simulink model "MMC_9lvl_matriz_tri_v12_Renner"  (R2025a)
settings: Solver=FixedStepAuto  StartTime=0.0  StopTime=5  FixedStep=0.0000005  MaxStep=1e-6  RelTol=1e-3
InitFcn:
  | C=4000e-6;
  | Larm=15e-3;
  | Rarm=0;
  | R=5;
  | L=100e-6;
  | Vcc=250;
  | Vsm=Vcc*2/4;
  | Vcap0=Vsm;
  | FR=20000;
  | TS=1/FR; %0.00005 = 50 microsec
  | Vsa=120;
  | Pref=3000;
  | Qref=0;
libraries: spsIGBTDiodeLib x48, spsVoltageMeasurementLib x34, spsSeriesRLCBranchLib x33, spsCurrentMeasurementLib x10, spsGroundLib x4, spsACVoltageSourceLib x3, SignalEditorBlockLib x2, spsDCVoltageSourceLib x2, spsPowerLib x1, sps_lib x1
(part 1 of 2)
settings Model: Creator=bernardo  LastModifiedBy=renner
settings SolverCC: ZeroCrossAlgorithm=Adaptive  AlgebraicLoopSolver=TrustRegion
settings DataIOCC: ReturnWorkspaceOutputs=off
settings OptimizationCC: ReuseModelBlockBuffer=off
settings DebuggingCC: IgnoredZcDiagnostic=none  UnconnectedInputMsg=warning  UnconnectedOutputMsg=warning  UnconnectedLineMsg=warning  ArithmeticOperatorsInVariantConditions=warning
settings ModelReferenceCC: EnableRefExpFcnMdlSchedulingChecks=on
settings SFSimCC: SimUseLocalCustomCode=off  CustomCodeUndefinedFunction=UseInterfaceOnly
settings RTWCC: RTWUseLocalCustomCode=off  GPUComputeCapability=3.5

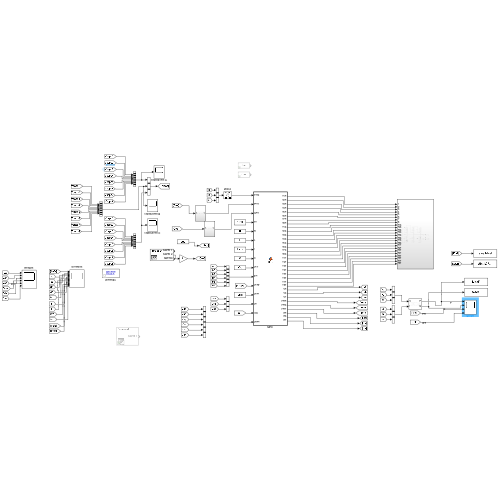
[thumbnail: Simulink's stored preview of the top-level diagram]
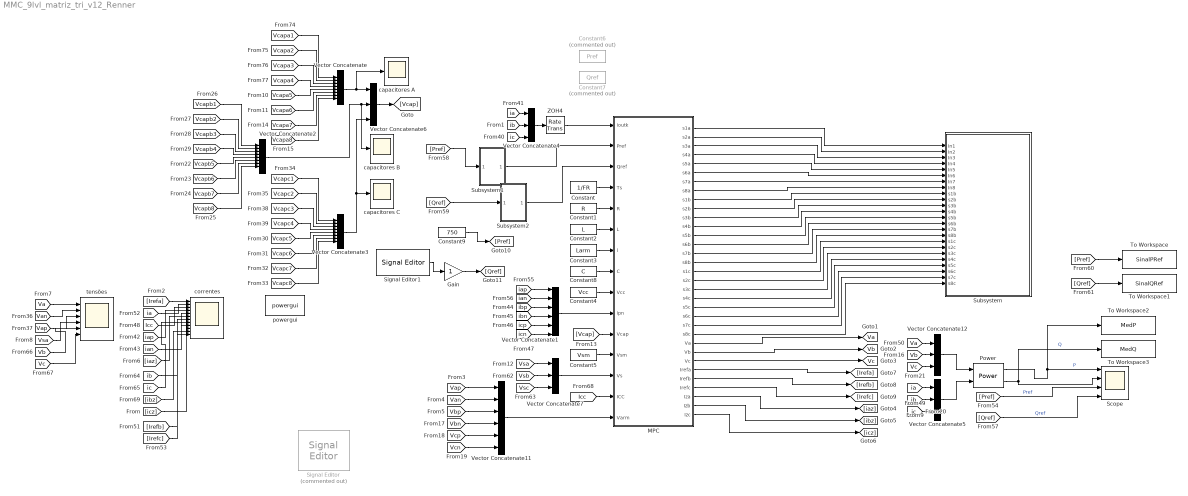
== system MMC_9lvl_matriz_tri_v12_Renner ==
  Constant : Constant  Value=1/FR
  Constant1 : Constant  Value=R
  Constant2 : Constant  Value=L
  Constant3 : Constant  Value=Larm
  Constant4 : Constant  Value=Vcc
  Constant5 : Constant  Value=Vsm
  Constant6 : Constant  Commented=on  Value=Pref
  Constant7 : Constant  Commented=on  Value=Qref
  Constant8 : Constant  Value=C
  Constant9 : Constant  Value=750
  Gain : Gain
  MPC : MATLAB Function  TreatAsAtomicUnit=on  SystemSampleTime=0.00005
  Power : spsPowerLib/Power  Freq=60  Vinit=[1, 0]  Iinit=[1, 0]  Ts=0
  Scope : Scope  NumInputPorts=4
      settings: ActiveDisplayYMinimum=-323.77012117483849  ActiveDisplayYMaximum=2913.931090573547
  Signal Editor : SignalEditorBlockLib/Signal Editor  Commented=on  FileName=G:\My Drive\PESQUISA\SIMULACOES\sinais.mat  ActiveScenario=Scenario2  ActiveSignal=Steps Q  IsBus=off  OutputBusObjectStr=Bus: BusObject  SampleTime=0  Interpolate=off  ZeroCross=off  OutputAfterFinalValue=Setting to zero  Unit=inherit  PreserveSignalName=on  ApplySigPropsToAllScenarios=on  ApplySigPropsToAllSignals=on  SignalPropertySource=Dialog parameters
  Signal Editor1 : SignalEditorBlockLib/Signal Editor  FileName=/Users/renner/Downloads/Sinais.mat  ActiveScenario=Scenario  ActiveSignal=Signal 2  IsBus=off  OutputBusObjectStr=Bus: BusObject  SampleTime=0  ZeroCross=off  OutputAfterFinalValue=Setting to zero  Unit=inherit  PreserveSignalName=on  ApplySigPropsToAllScenarios=on  ApplySigPropsToAllSignals=off  SignalPropertySource=Dialog parameters
  Subsystem : Subsystem
  Subsystem1 : Subsystem
  Subsystem2 : Subsystem
  To Workspace : ToWorkspace  VariableName=SinalPRef  SampleTime=0.0005
      settings: Decimation=3  Save2DSignal=2-D array (concatenate along first dimension)
  To Workspace1 : ToWorkspace  VariableName=SinalQRef  SampleTime=0.0005
      settings: Decimation=3  Save2DSignal=2-D array (concatenate along first dimension)
  To Workspace2 : ToWorkspace  VariableName=MedP  SampleTime=0.0005
      settings: Decimation=3  Save2DSignal=2-D array (concatenate along first dimension)
  To Workspace3 : ToWorkspace  VariableName=MedQ  SampleTime=0.0005
      settings: Decimation=3  Save2DSignal=2-D array (concatenate along first dimension)
  Vector Concatenate : Concatenate  NumInputs=8
  Vector Concatenate1 : Concatenate  NumInputs=6
  Vector Concatenate11 : Concatenate  NumInputs=6
  Vector Concatenate{4..7,12} (5 alike) : Concatenate  NumInputs=3
  Vector Concatenate2 : Concatenate  NumInputs=8
  Vector Concatenate3 : Concatenate  NumInputs=8
  ZOH4 : RateTransition  OutPortSampleTime=TS
  capacitores A : Scope
      settings: ActiveDisplayYMinimum=96.83935  ActiveDisplayYMaximum=130.64864
  capacitores B : Scope
      settings: ActiveDisplayYMinimum=97.09716  ActiveDisplayYMaximum=129.55775  DataLoggingVariableName=ScopeData2
  capacitores C : Scope
      settings: ActiveDisplayYMinimum=97.83131  ActiveDisplayYMaximum=129.00851  DataLoggingVariableName=ScopeData3
  correntes : Scope  NumInputPorts=12
      settings: ActiveDisplayYMinimum=-28.003686399512119  ActiveDisplayYMaximum=28.003686399512119
  powergui : sps_lib/powergui  Priority=1  SimulationMode=Discrete  SampleTime=0.00005  frequency=60  Iterations=50  frequencyindice=0  Pbase=100e6  ErrMax=1e-4  UnitsV=kV  UnitsW=MW  buscounter=0  FunctionMessages=off  echomessages=off  EnableUseOfTLC=off  CurrentSourceSwitches=off  DisableSnubberDevices=off  DisableRonSwitches=off  DisableVfSwitches=off  DisplayEquations=off  AutomaticDiscreteSolvers=off  SolverType=Tustin/Backward Euler (TBE)  Interpol=off  ExternalGateDelay=off  methode=off  Ts=100  x0status=blocks  SPID=on  SwTol=0  HookPort=off  NonlinearTolerance=1e-4  nMaxIteration=100  ContinueOnMaxIteration=off  RestoreLinks=warning  ResistiveCurrentMeasurement=off  Frange=[0:2:500]  Ylog=off  Xlog=on  ShowGrid=off  save=off  variable=ZData  structure=Scope1  ZoomFFT=off  StartTime=0.0  cycles=10  DisplayStyle=2  fundamental=60  FreqAxis=off  MaxFrequency=20000  frequencyindicesteady=1  RmsSteady=1  display=off
  tensões : Scope  NumInputPorts=6
      settings: ActiveDisplayYMinimum=-296.50571696969695  ActiveDisplayYMaximum=516.307633030303  DataLoggingVariableName=ScopeData2
  tag scope: Va=global, Vb=global, Vc=global
  wires:
  Constant1/1 -> MPC/5(R)
  Constant/1 -> MPC/4(Ts)
  Constant3/1 -> MPC/7(l)
  Constant4/1 -> MPC/9(Vcc)
  Constant2/1 -> MPC/6(L)
  [iap] -> correntes/4
  [ian] -> correntes/5
  [Icc] -> correntes/3
  [ia] -> correntes/2
  [Van] -> tensões/2
  [Vcapa1] -> Vector Concatenate/1
  [Vcapa2] -> Vector Concatenate/2
  [Vcapa3] -> Vector Concatenate/3
  [Vcapa4] -> Vector Concatenate/4
  [iap] -> Vector Concatenate1/1
  [ian] -> Vector Concatenate1/2
  Vector Concatenate1/1 -> MPC/10(ipn)
  [Vap] -> tensões/3
  [Vcapa5] -> Vector Concatenate/5
  [Vcapa6] -> Vector Concatenate/6
  [Vcapa7] -> Vector Concatenate/7
  [Vcapa8] -> Vector Concatenate/8
  [Irefa] -> correntes/1
  [iaz] -> correntes/6
  MPC/1(s1a) -> Subsystem/1(In1)
  MPC/2(s2a) -> Subsystem/2(In2)
  MPC/3(s3a) -> Subsystem/3(In3)
  MPC/4(s4a) -> Subsystem/4(In4)
  MPC/5(s5a) -> Subsystem/5(In5)
  MPC/6(s6a) -> Subsystem/6(In6)
  MPC/7(s7a) -> Subsystem/7(In7)
  MPC/8(s8a) -> Subsystem/8(In8)
  Constant5/1 -> MPC/12(Vsm)
  [Vsa] -> tensões/4
  [Va] -> tensões/1
  [Vcap] -> MPC/11(Vcap)
  Vector Concatenate2/1 -> capacitores B/1, Vector Concatenate6/2
  [Vcapb7] -> Vector Concatenate2/7
  [Vcapb5] -> Vector Concatenate2/5
  [Vcapb6] -> Vector Concatenate2/6
  [Vcapb3] -> Vector Concatenate2/3
  [Vcapb1] -> Vector Concatenate2/1
  [Vcapb2] -> Vector Concatenate2/2
  [Vcapb8] -> Vector Concatenate2/8
  [Vcapb4] -> Vector Concatenate2/4
  [Vcapc6] -> Vector Concatenate3/6
  [Vcapc4] -> Vector Concatenate3/4
  [Vcapc3] -> Vector Concatenate3/3
  [Vcapc1] -> Vector Concatenate3/1
  [Vcapc2] -> Vector Concatenate3/2
  [Vcapc8] -> Vector Concatenate3/8
  [Vcapc5] -> Vector Concatenate3/5
  Vector Concatenate3/1 -> Vector Concatenate6/3, capacitores C/1
  [Vcapc7] -> Vector Concatenate3/7
  MPC/9(s1b) -> Subsystem/9(s1b)
  MPC/10(s2b) -> Subsystem/10(s2b)
  MPC/11(s3b) -> Subsystem/11(s3b)
  MPC/12(s4b) -> Subsystem/12(s4b)
  MPC/13(s5b) -> Subsystem/13(s5b)
  MPC/14(s6b) -> Subsystem/14(s6b)
  MPC/15(s7b) -> Subsystem/15(s7b)
  MPC/16(s8b) -> Subsystem/16(s8b)
  MPC/17(s1c) -> Subsystem/17(s1c)
  MPC/18(s2c) -> Subsystem/18(s2c)
  MPC/19(s3c) -> Subsystem/19(s3c)
  MPC/20(s4c) -> Subsystem/20(s4c)
  MPC/21(s5c) -> Subsystem/21(s5c)
  MPC/22(s6c) -> Subsystem/22(s6c)
  MPC/23(s7c) -> Subsystem/23(s7c)
  MPC/24(s8c) -> Subsystem/24(s8c)
  [ia] -> Vector Concatenate4/1
  [ib] -> Vector Concatenate4/2
  [ic] -> Vector Concatenate4/3
  Vector Concatenate4/1 -> ZOH4/1
  ZOH4/1 -> MPC/1(ioutk)
  [ibp] -> Vector Concatenate1/3
  [ibn] -> Vector Concatenate1/4
  [icp] -> Vector Concatenate1/5
  [icn] -> Vector Concatenate1/6
  Vector Concatenate/1 -> capacitores A/1, Vector Concatenate6/1
  Vector Concatenate6/1 -> [Vcap]
  [Vsc] -> Vector Concatenate7/3
  [ib] -> correntes/7
  [ic] -> correntes/8
  [Vb] -> tensões/5
  [Vc] -> tensões/6
  [Icc] -> MPC/14(ICC)
  [ibz] -> correntes/9
  [icz] -> correntes/10
  [Vap] -> Vector Concatenate11/1
  [Van] -> Vector Concatenate11/2
  [Vbp] -> Vector Concatenate11/3
  [Vbn] -> Vector Concatenate11/4
  [Vcp] -> Vector Concatenate11/5
  [Vcn] -> Vector Concatenate11/6
  Vector Concatenate11/1 -> MPC/15(Varm)
  Vector Concatenate7/1 -> MPC/13(Vs)
  [Vsa] -> Vector Concatenate7/1
  [Vsb] -> Vector Concatenate7/2
  MPC/25(Va) -> [Va]
  MPC/26(Vb) -> [Vb]
  MPC/27(Vc) -> [Vc]
  MPC/28(Irefa) -> [Irefa]
  MPC/29(Irefb) -> [Irefb]
  MPC/30(Irefc) -> [Irefc]
  MPC/31(Iza) -> [iaz]
  MPC/32(Izb) -> [ibz]
  MPC/33(Izc) -> [icz]
  [ia] -> Vector Concatenate5/1
  [ic] -> Vector Concatenate5/3
  [Vb] -> Vector Concatenate12/2
  [Vc] -> Vector Concatenate12/3
  [Va] -> Vector Concatenate12/1
  [ib] -> Vector Concatenate5/2
  [Irefb] -> correntes/11
  [Irefc] -> correntes/12
  Constant8/1 -> MPC/8(C)
  Power/1 -> Scope/1, To Workspace2/1  "P"
  Power/2 -> Scope/2, To Workspace3/1  "Q"
  Vector Concatenate12/1 -> Power/1
  Vector Concatenate5/1 -> Power/2
  [Qref] -> Subsystem2/1(In1)
  [Pref] -> To Workspace/1
  [Qref] -> To Workspace1/1
  [Pref] -> Subsystem1/1(In1)
  Subsystem1/1(Out1) -> MPC/2(Pref)
  [Pref] -> Scope/3  "Pref"
  Constant9/1 -> [Pref]
  [Qref] -> Scope/4  "Qref"
  Gain/1 -> [Qref]
  Subsystem2/1(Out1) -> MPC/3(Qref)
  Signal Editor1/2 -> Gain/1

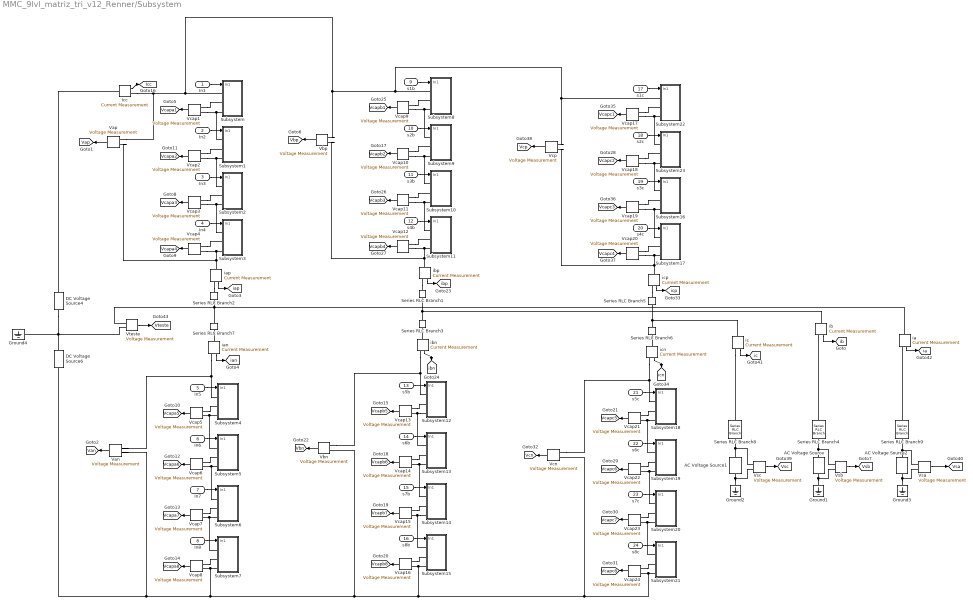
== system MMC_9lvl_matriz_tri_v12_Renner/Subsystem ==
  In1 : Inport
  In2 : Inport  Port=2
  In3 : Inport  Port=3
  In4 : Inport  Port=4
  In5 : Inport  Port=5
  In6 : Inport  Port=6
  In7 : Inport  Port=7
  In8 : Inport  Port=8
  s1b : Inport  Port=9
  s2b : Inport  Port=10
  s3b : Inport  Port=11
  s4b : Inport  Port=12
  s5b : Inport  Port=13
  s6b : Inport  Port=14
  s7b : Inport  Port=15
  s8b : Inport  Port=16
  s1c : Inport  Port=17
  s2c : Inport  Port=18
  s3c : Inport  Port=19
  s4c : Inport  Port=20
  s5c : Inport  Port=21
  s6c : Inport  Port=22
  s7c : Inport  Port=23
  s8c : Inport  Port=24
  AC Voltage Source : spsACVoltageSourceLib/AC Voltage Source  Amplitude=Vsa  Phase=-120  Frequency=60  SampleTime=0  Measurements=None  BusType=swing  Pref=10e3  Qref=0  Qmin=-inf  Qmax=+inf
  AC Voltage Source1 : spsACVoltageSourceLib/AC Voltage Source  Amplitude=Vsa  Phase=120  Frequency=60  SampleTime=0  Measurements=None  BusType=swing  Pref=10e3  Qref=0  Qmin=-inf  Qmax=+inf
  AC Voltage Source2 : spsACVoltageSourceLib/AC Voltage Source  Amplitude=Vsa  Phase=0  Frequency=60  SampleTime=0  Measurements=None  BusType=swing  Pref=10e3  Qref=0  Qmin=-inf  Qmax=+inf
  DC Voltage Source4 : spsDCVoltageSourceLib/DC Voltage Source  Amplitude=Vcc  Measurements=None
  DC Voltage Source6 : spsDCVoltageSourceLib/DC Voltage Source  Amplitude=Vcc  Measurements=None
  Ground{1..4} (4 alike) : spsGroundLib/Ground  LConnTagsString=a
  Icc : spsCurrentMeasurementLib/Current Measurement  PhasorSimulation=off  OutputType=Magnitude  PSBequivalent=0
  Series RLC Branch{1..3,5..7} (6 alike) : spsSeriesRLCBranchLib/Series RLC Branch  LConnTagsString=__new0  RConnTagsString=__new0  BranchType=L  Resistance=0  Inductance=Larm  SetiL0=off  InitialCurrent=0  Capacitance=0  Setx0=off  InitialVoltage=0  Measurements=None
  Series RLC Branch4 : spsSeriesRLCBranchLib/Series RLC Branch  LConnTagsString=__new0  RConnTagsString=__new0  BranchType=RL  Resistance=R  Inductance=L  SetiL0=off  InitialCurrent=0  Capacitance=1e-6  Setx0=off  InitialVoltage=0  Measurements=None
  Series RLC Branch8 : spsSeriesRLCBranchLib/Series RLC Branch  LConnTagsString=__new0  RConnTagsString=__new0  BranchType=RL  Resistance=R  Inductance=L  SetiL0=off  InitialCurrent=0  Capacitance=1e-6  Setx0=off  InitialVoltage=0  Measurements=None
  Series RLC Branch9 : spsSeriesRLCBranchLib/Series RLC Branch  LConnTagsString=__new0  RConnTagsString=__new0  BranchType=RL  Resistance=R  Inductance=L  SetiL0=off  InitialCurrent=0  Capacitance=1e-6  Setx0=off  InitialVoltage=0  Measurements=None
  Subsystem : Subsystem
  Subsystem1 : Subsystem
  Subsystem10 : Subsystem
  Subsystem11 : Subsystem
  Subsystem12 : Subsystem
  Subsystem13 : Subsystem
  Subsystem14 : Subsystem
  Subsystem15 : Subsystem
  Subsystem16 : Subsystem
  Subsystem17 : Subsystem
  Subsystem18 : Subsystem
  Subsystem19 : Subsystem
  Subsystem2 : Subsystem
  Subsystem20 : Subsystem
  Subsystem21 : Subsystem
  Subsystem22 : Subsystem
  Subsystem23 : Subsystem
  Subsystem3 : Subsystem
  Subsystem4 : Subsystem
  Subsystem5 : Subsystem
  Subsystem6 : Subsystem
  Subsystem7 : Subsystem
  Subsystem8 : Subsystem
  Subsystem9 : Subsystem
  Van : spsVoltageMeasurementLib/Voltage Measurement  PhasorSimulation=off  OutputType=Complex  PSBequivalent=0
  Vap : spsVoltageMeasurementLib/Voltage Measurement  PhasorSimulation=off  OutputType=Complex  PSBequivalent=0
  Vbn : spsVoltageMeasurementLib/Voltage Measurement  PhasorSimulation=off  OutputType=Complex  PSBequivalent=0
  Vbp : spsVoltageMeasurementLib/Voltage Measurement  PhasorSimulation=off  OutputType=Complex  PSBequivalent=0
  Vcap{1..24} (24 alike) : spsVoltageMeasurementLib/Voltage Measurement  PhasorSimulation=off  OutputType=Complex  PSBequivalent=0
  Vcn : spsVoltageMeasurementLib/Voltage Measurement  PhasorSimulation=off  OutputType=Complex  PSBequivalent=0
  Vcp : spsVoltageMeasurementLib/Voltage Measurement  PhasorSimulation=off  OutputType=Complex  PSBequivalent=0
  Vsa : spsVoltageMeasurementLib/Voltage Measurement  PhasorSimulation=off  OutputType=Complex  PSBequivalent=0
  Vsb : spsVoltageMeasurementLib/Voltage Measurement  PhasorSimulation=off  OutputType=Complex  PSBequivalent=0
  Vsc : spsVoltageMeasurementLib/Voltage Measurement  PhasorSimulation=off  OutputType=Complex  PSBequivalent=0
  Vteste : spsVoltageMeasurementLib/Voltage Measurement  PhasorSimulation=off  OutputType=Complex  PSBequivalent=0
  ia : spsCurrentMeasurementLib/Current Measurement  PhasorSimulation=off  OutputType=Magnitude  PSBequivalent=0
  ian : spsCurrentMeasurementLib/Current Measurement  PhasorSimulation=off  OutputType=Magnitude  PSBequivalent=0
  iap : spsCurrentMeasurementLib/Current Measurement  PhasorSimulation=off  OutputType=Magnitude  PSBequivalent=0
  ib : spsCurrentMeasurementLib/Current Measurement  PhasorSimulation=off  OutputType=Magnitude  PSBequivalent=0
  ibn : spsCurrentMeasurementLib/Current Measurement  PhasorSimulation=off  OutputType=Magnitude  PSBequivalent=0
  ibp : spsCurrentMeasurementLib/Current Measurement  PhasorSimulation=off  OutputType=Magnitude  PSBequivalent=0
  ic : spsCurrentMeasurementLib/Current Measurement  PhasorSimulation=off  OutputType=Magnitude  PSBequivalent=0
  icn : spsCurrentMeasurementLib/Current Measurement  PhasorSimulation=off  OutputType=Magnitude  PSBequivalent=0
  icp : spsCurrentMeasurementLib/Current Measurement  PhasorSimulation=off  OutputType=Magnitude  PSBequivalent=0
  tag scope: Icc=global, Van=global, Vap=global, Vbn=global, Vbp=global, Vcapa1=global, Vcapa2=global, Vcapa3=global, Vcapa4=global, Vcapa5=global, Vcapa6=global, Vcapa7=global, Vcapa8=global, Vcapb1=global, Vcapb2=global, Vcapb3=global, Vcapb4=global, Vcapb5=global, Vcapb6=global, Vcapb7=global, Vcapb8=global, Vcapc1=global, Vcapc2=global, Vcapc3=global, Vcapc4=global, Vcapc5=global, Vcapc6=global, Vcapc7=global, Vcapc8=global, Vcn=global, Vcp=global, Vsa=global, Vsb=global, Vsc=global, Vteste=global, ia=global, ian=global, iap=global, ib=global, ibn=global, ibp=global, ic=global, icn=global, icp=global
  wires:
  ib/1 -> [ib]
  Van/1 -> [Van]
  iap/1 -> [iap]
  ian/1 -> [ian]
  Vcap1/1 -> [Vcapa1]
  In1/1 -> Subsystem/1(In1)
  In2/1 -> Subsystem1/1(In1)
  Vcap2/1 -> [Vcapa2]
  Vcap3/1 -> [Vcapa3]
  In3/1 -> Subsystem2/1(In1)
  In4/1 -> Subsystem3/1(In1)
  Vcap4/1 -> [Vcapa4]
  In5/1 -> Subsystem4/1(In1)
  Vcap5/1 -> [Vcapa5]
  Vap/1 -> [Vap]
  Vcap6/1 -> [Vcapa6]
  In6/1 -> Subsystem5/1(In1)
  In8/1 -> Subsystem7/1(In1)
  Vcap8/1 -> [Vcapa8]
  Vcap7/1 -> [Vcapa7]
  In7/1 -> Subsystem6/1(In1)
  Icc/1 -> [Icc]
  Vsb/1 -> [Vsb]
  s6b/1 -> Subsystem13/1(In1)
  s5b/1 -> Subsystem12/1(In1)
  ibn/1 -> [ibn]
  Vcap12/1 -> [Vcapb4]
  Vcap16/1 -> [Vcapb8]
  s2b/1 -> Subsystem9/1(In1)
  s8b/1 -> Subsystem15/1(In1)
  Vcap13/1 -> [Vcapb5]
  ibp/1 -> [ibp]
  Vcap10/1 -> [Vcapb2]
  s4b/1 -> Subsystem11/1(In1)
  s7b/1 -> Subsystem14/1(In1)
  Vbp/1 -> [Vbp]
  s1b/1 -> Subsystem8/1(In1)
  s3b/1 -> Subsystem10/1(In1)
  Vbn/1 -> [Vbn]
  Vcap14/1 -> [Vcapb6]
  Vcap9/1 -> [Vcapb1]
  Vcap15/1 -> [Vcapb7]
  Vcap11/1 -> [Vcapb3]
  Vcap19/1 -> [Vcapc3]
  Vcap22/1 -> [Vcapc6]
  s3c/1 -> Subsystem16/1(In1)
  Vcap23/1 -> [Vcapc7]
  Vcp/1 -> [Vcp]
  Vcap21/1 -> [Vcapc5]
  s7c/1 -> Subsystem20/1(In1)
  Vcap17/1 -> [Vcapc1]
  s6c/1 -> Subsystem19/1(In1)
  icn/1 -> [icn]
  s8c/1 -> Subsystem21/1(In1)
  s2c/1 -> Subsystem23/1(In1)
  s5c/1 -> Subsystem18/1(In1)
  s4c/1 -> Subsystem17/1(In1)
  icp/1 -> [icp]
  Vcap18/1 -> [Vcapc2]
  Vcap20/1 -> [Vcapc4]
  Vcap24/1 -> [Vcapc8]
  s1c/1 -> Subsystem22/1(In1)
  Vcn/1 -> [Vcn]
  Vsc/1 -> [Vsc]
  Vsa/1 -> [Vsa]
  ia/1 -> [ia]
  ic/1 -> [ic]
  Vteste/1 -> [Vteste]
  connections:
  Vcap1/LConn2 -- Subsystem1/LConn1 -- Subsystem/LConn3
  Vcap1/LConn1 -- Subsystem/LConn2
  Vcap2/LConn1 -- Subsystem1/LConn2
  Vcap2/LConn2 -- Subsystem2/LConn1 -- Subsystem1/LConn3
  Vcap3/LConn2 -- Subsystem3/LConn1 -- Subsystem2/LConn3
  Vcap3/LConn1 -- Subsystem2/LConn2
  Vcap4/LConn2 -- Vap/LConn2 -- iap/LConn1 -- Subsystem3/LConn3
  Vcap4/LConn1 -- Subsystem3/LConn2
  Icc/LConn1 -- DC Voltage Source4/RConn1
  iap/RConn1 -- Series RLC Branch2/RConn1
  Series RLC Branch7/RConn1 -- Vteste/LConn1 -- ia/LConn1 -- Series RLC Branch2/LConn1
  Series RLC Branch4/LConn1 -- ib/RConn1
  ian/LConn1 -- Series RLC Branch7/LConn1
  ian/RConn1 -- Van/LConn1 -- Subsystem4/LConn1
  Vcap5/LConn2 -- Subsystem5/LConn1 -- Subsystem4/LConn3
  Vcap5/LConn1 -- Subsystem4/LConn2
  Vcap6/LConn1 -- Subsystem5/LConn2
  Vcap6/LConn2 -- Subsystem6/LConn1 -- Subsystem5/LConn3
  Subsystem7/LConn1 -- Vcap7/LConn2 -- Subsystem6/LConn3
  Subsystem21/LConn3 -- Vcap24/LConn2 -- Vbn/LConn2 -- DC Voltage Source6/LConn1 -- Van/LConn2 -- Vcap8/LConn2 -- Subsystem7/LConn3 -- Vcap16/LConn2 -- Subsystem15/LConn3 -- Vcn/LConn2
  Vcap8/LConn1 -- Subsystem7/LConn2
  Vcap7/LConn1 -- Subsystem6/LConn2
  Vcp/LConn1 -- Vbp/LConn1 -- Vap/LConn1 -- Icc/RConn1 -- Subsystem/LConn1 -- Subsystem8/LConn1 -- Subsystem22/LConn1
  Ground4/LConn1 -- DC Voltage Source4/LConn1 -- Vteste/LConn2 -- DC Voltage Source6/RConn1
  AC Voltage Source/RConn1 -- Vsb/LConn1 -- Series RLC Branch4/RConn1
  Ground1/LConn1 -- AC Voltage Source/LConn1 -- Vsb/LConn2
  Subsystem10/LConn3 -- Vcap11/LConn2 -- Subsystem11/LConn1
  Subsystem11/LConn3 -- Vcap12/LConn2 -- Vbp/LConn2 -- ibp/LConn1
  Subsystem12/LConn1 -- ibn/RConn1 -- Vbn/LConn1
  Subsystem12/LConn3 -- Vcap13/LConn2 -- Subsystem13/LConn1
  Series RLC Branch3/RConn1 -- ib/LConn1 -- Series RLC Branch1/LConn1
  Subsystem9/LConn3 -- Vcap10/LConn2 -- Subsystem10/LConn1
  Subsystem8/LConn3 -- Vcap9/LConn2 -- Subsystem9/LConn1
  Subsystem13/LConn3 -- Vcap14/LConn2 -- Subsystem14/LConn1
  Subsystem14/LConn3 -- Subsystem15/LConn1 -- Vcap15/LConn2
  Vcap11/LConn1 -- Subsystem10/LConn2
  Vcap15/LConn1 -- Subsystem14/LConn2
  ibn/LConn1 -- Series RLC Branch3/LConn1
  ibp/RConn1 -- Series RLC Branch1/RConn1
  Vcap12/LConn1 -- Subsystem11/LConn2
  Vcap9/LConn1 -- Subsystem8/LConn2
  Vcap10/LConn1 -- Subsystem9/LConn2
  Vcap14/LConn1 -- Subsystem13/LConn2
  Vcap16/LConn1 -- Subsystem15/LConn2
  Vcap13/LConn1 -- Subsystem12/LConn2
  Subsystem19/LConn3 -- Vcap22/LConn2 -- Subsystem20/LConn1
  Subsystem22/LConn3 -- Vcap17/LConn2 -- Subsystem23/LConn1
  Subsystem20/LConn3 -- Subsystem21/LConn1 -- Vcap23/LConn2
  ic/RConn1 -- Series RLC Branch8/LConn1
  Subsystem18/LConn3 -- Vcap21/LConn2 -- Subsystem19/LConn1
  Subsystem18/LConn1 -- icn/RConn1 -- Vcn/LConn1
  Subsystem17/LConn3 -- Vcap20/LConn2 -- Vcp/LConn2 -- icp/LConn1
  Subsystem16/LConn3 -- Vcap19/LConn2 -- Subsystem17/LConn1
  Subsystem23/LConn3 -- Vcap18/LConn2 -- Subsystem16/LConn1
  Vcap21/LConn1 -- Subsystem18/LConn2
  Vcap18/LConn1 -- Subsystem23/LConn2
  Vcap24/LConn1 -- Subsystem21/LConn2
  Vcap17/LConn1 -- Subsystem22/LConn2
  Vcap22/LConn1 -- Subsystem19/LConn2
  Vcap20/LConn1 -- Subsystem17/LConn2
  Vcap23/LConn1 -- Subsystem20/LConn2
  icn/LConn1 -- Series RLC Branch6/LConn1
  icp/RConn1 -- Series RLC Branch5/RConn1
  Vcap19/LConn1 -- Subsystem16/LConn2
  AC Voltage Source1/RConn1 -- Vsc/LConn1 -- Series RLC Branch8/RConn1
  Ground2/LConn1 -- AC Voltage Source1/LConn1 -- Vsc/LConn2
  AC Voltage Source2/RConn1 -- Vsa/LConn1 -- Series RLC Branch9/RConn1
  Ground3/LConn1 -- AC Voltage Source2/LConn1 -- Vsa/LConn2
  Series RLC Branch9/LConn1 -- ia/RConn1
  Series RLC Branch6/RConn1 -- ic/LConn1 -- Series RLC Branch5/LConn1

== system MMC_9lvl_matriz_tri_v12_Renner/Subsystem1 ==
  In1 : Inport
  Fcn : Fcn  Expr=((44.38019/sqrt(u))+0.75116)*u
  Fcn1 : Fcn  Expr=((29.2367/u)-(1.520184/sqrt(u))+1.0009)*u
  Out1 : Outport
  wires:
  In1/1 -> Fcn/1
  Fcn/1 -> Fcn1/1
  Fcn1/1 -> Out1/1

== system MMC_9lvl_matriz_tri_v12_Renner/Subsystem2 ==
  In1 : Inport
  Fcn : Fcn  Expr=((-931.5321/u)+(67.9151/(sqrt(u)))+0.8719)*u
  Out1 : Outport
  wires:
  In1/1 -> Fcn/1
  Fcn/1 -> Out1/1

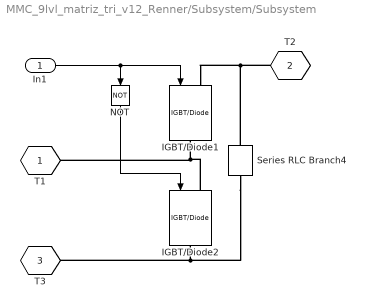
== system MMC_9lvl_matriz_tri_v12_Renner/Subsystem/Subsystem ==
  In1 : Inport
  IGBT/Diode1 : spsIGBTDiodeLib/IGBT//Diode  Ron=1e-3  Rs=1e8  Cs=inf  Measurements=off
  IGBT/Diode2 : spsIGBTDiodeLib/IGBT//Diode  Ron=1e-3  Rs=1e8  Cs=inf  Measurements=off
  NOT : Logic  Operator=NOT  IconShape=distinctive  AllPortsSameDT=off  OutDataTypeStr=boolean
  Series RLC Branch4 : spsSeriesRLCBranchLib/Series RLC Branch  LConnTagsString=__new0  RConnTagsString=__new0  BranchType=C  Resistance=R  Inductance=L  SetiL0=off  InitialCurrent=0  Capacitance=C  Setx0=on  InitialVoltage=Vcap0  Measurements=None
  T1 : PMIOPort  Tag=PMCPort  Side=Left
  T2 : PMIOPort  Tag=PMCPort  Port=2  Side=Left
  T3 : PMIOPort  Tag=PMCPort  Port=3  Side=Left
  wires:
  NOT/1 -> IGBT/Diode2/1
  In1/1 -> NOT/1, IGBT/Diode1/1
  connections:
  Series RLC Branch4/RConn1 -- T3/RConn1 -- IGBT/Diode2/RConn1
  IGBT/Diode2/LConn1 -- IGBT/Diode1/RConn1 -- T1/RConn1
  Series RLC Branch4/LConn1 -- T2/RConn1 -- IGBT/Diode1/LConn1

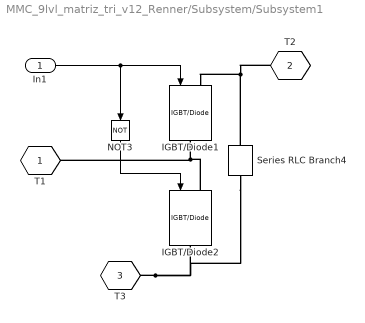
== system MMC_9lvl_matriz_tri_v12_Renner/Subsystem/Subsystem1 ==
  In1 : Inport
  IGBT/Diode1 : spsIGBTDiodeLib/IGBT//Diode  Ron=1e-3  Rs=1e8  Cs=inf  Measurements=off
  IGBT/Diode2 : spsIGBTDiodeLib/IGBT//Diode  Ron=1e-3  Rs=1e8  Cs=inf  Measurements=off
  NOT3 : Logic  Operator=NOT  IconShape=distinctive  AllPortsSameDT=off  OutDataTypeStr=boolean
  Series RLC Branch4 : spsSeriesRLCBranchLib/Series RLC Branch  LConnTagsString=__new0  RConnTagsString=__new0  BranchType=C  Resistance=R  Inductance=L  SetiL0=off  InitialCurrent=0  Capacitance=C  Setx0=on  InitialVoltage=Vcap0  Measurements=None
  T1 : PMIOPort  Tag=PMCPort  Side=Left
  T2 : PMIOPort  Tag=PMCPort  Port=2  Side=Left
  T3 : PMIOPort  Tag=PMCPort  Port=3  Side=Left
  wires:
  NOT3/1 -> IGBT/Diode2/1
  In1/1 -> NOT3/1, IGBT/Diode1/1
  connections:
  T3/RConn1 -- Series RLC Branch4/RConn1 -- IGBT/Diode2/RConn1
  IGBT/Diode2/LConn1 -- IGBT/Diode1/RConn1 -- T1/RConn1
  T2/RConn1 -- Series RLC Branch4/LConn1 -- IGBT/Diode1/LConn1

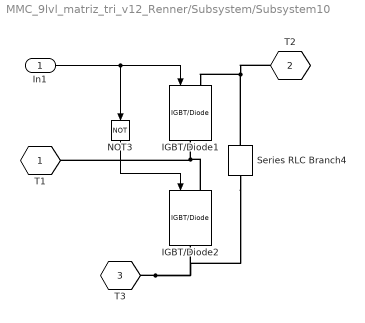
== system MMC_9lvl_matriz_tri_v12_Renner/Subsystem/Subsystem10 ==
  In1 : Inport
  IGBT/Diode1 : spsIGBTDiodeLib/IGBT//Diode  Ron=1e-3  Rs=1e8  Cs=inf  Measurements=off
  IGBT/Diode2 : spsIGBTDiodeLib/IGBT//Diode  Ron=1e-3  Rs=1e8  Cs=inf  Measurements=off
  NOT3 : Logic  Operator=NOT  IconShape=distinctive  AllPortsSameDT=off  OutDataTypeStr=boolean
  Series RLC Branch4 : spsSeriesRLCBranchLib/Series RLC Branch  LConnTagsString=__new0  RConnTagsString=__new0  BranchType=C  Resistance=R  Inductance=L  SetiL0=off  InitialCurrent=0  Capacitance=C  Setx0=on  InitialVoltage=Vcap0  Measurements=None
  T1 : PMIOPort  Tag=PMCPort  Side=Left
  T2 : PMIOPort  Tag=PMCPort  Port=2  Side=Left
  T3 : PMIOPort  Tag=PMCPort  Port=3  Side=Left
  wires:
  NOT3/1 -> IGBT/Diode2/1
  In1/1 -> NOT3/1, IGBT/Diode1/1
  connections:
  T3/RConn1 -- Series RLC Branch4/RConn1 -- IGBT/Diode2/RConn1
  IGBT/Diode2/LConn1 -- IGBT/Diode1/RConn1 -- T1/RConn1
  T2/RConn1 -- Series RLC Branch4/LConn1 -- IGBT/Diode1/LConn1

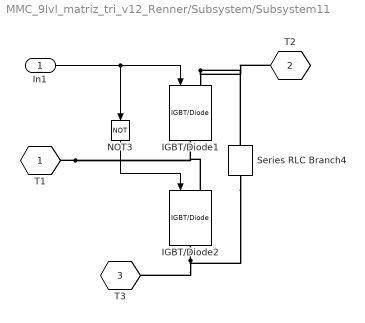
== system MMC_9lvl_matriz_tri_v12_Renner/Subsystem/Subsystem11 ==
  In1 : Inport
  IGBT/Diode1 : spsIGBTDiodeLib/IGBT//Diode  Ron=1e-3  Rs=1e8  Cs=inf  Measurements=off
  IGBT/Diode2 : spsIGBTDiodeLib/IGBT//Diode  Ron=1e-3  Rs=1e8  Cs=inf  Measurements=off
  NOT3 : Logic  Operator=NOT  IconShape=distinctive  AllPortsSameDT=off  OutDataTypeStr=boolean
  Series RLC Branch4 : spsSeriesRLCBranchLib/Series RLC Branch  LConnTagsString=__new0  RConnTagsString=__new0  BranchType=C  Resistance=R  Inductance=L  SetiL0=off  InitialCurrent=0  Capacitance=C  Setx0=on  InitialVoltage=Vcap0  Measurements=None
  T1 : PMIOPort  Tag=PMCPort  Side=Left
  T2 : PMIOPort  Tag=PMCPort  Port=2  Side=Left
  T3 : PMIOPort  Tag=PMCPort  Port=3  Side=Left
  wires:
  In1/1 -> IGBT/Diode1/1, NOT3/1
  NOT3/1 -> IGBT/Diode2/1
  connections:
  IGBT/Diode1/LConn1 -- Series RLC Branch4/LConn1 -- T2/RConn1
  T1/RConn1 -- IGBT/Diode1/RConn1 -- IGBT/Diode2/LConn1
  IGBT/Diode2/RConn1 -- Series RLC Branch4/RConn1 -- T3/RConn1

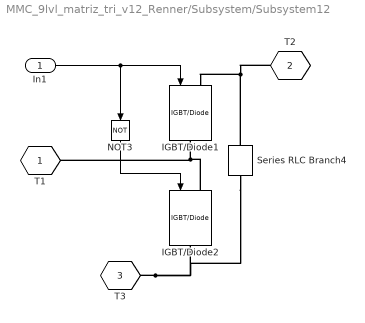
== system MMC_9lvl_matriz_tri_v12_Renner/Subsystem/Subsystem12 ==
  In1 : Inport
  IGBT/Diode1 : spsIGBTDiodeLib/IGBT//Diode  Ron=1e-3  Rs=1e8  Cs=inf  Measurements=off
  IGBT/Diode2 : spsIGBTDiodeLib/IGBT//Diode  Ron=1e-3  Rs=1e8  Cs=inf  Measurements=off
  NOT3 : Logic  Operator=NOT  IconShape=distinctive  AllPortsSameDT=off  OutDataTypeStr=boolean
  Series RLC Branch4 : spsSeriesRLCBranchLib/Series RLC Branch  LConnTagsString=__new0  RConnTagsString=__new0  BranchType=C  Resistance=R  Inductance=L  SetiL0=off  InitialCurrent=0  Capacitance=C  Setx0=on  InitialVoltage=Vcap0  Measurements=None
  T1 : PMIOPort  Tag=PMCPort  Side=Left
  T2 : PMIOPort  Tag=PMCPort  Port=2  Side=Left
  T3 : PMIOPort  Tag=PMCPort  Port=3  Side=Left
  wires:
  NOT3/1 -> IGBT/Diode2/1
  In1/1 -> NOT3/1, IGBT/Diode1/1
  connections:
  T3/RConn1 -- Series RLC Branch4/RConn1 -- IGBT/Diode2/RConn1
  IGBT/Diode2/LConn1 -- IGBT/Diode1/RConn1 -- T1/RConn1
  T2/RConn1 -- Series RLC Branch4/LConn1 -- IGBT/Diode1/LConn1

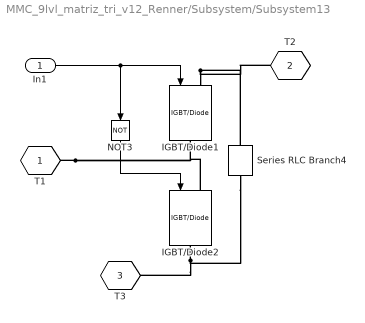
== system MMC_9lvl_matriz_tri_v12_Renner/Subsystem/Subsystem13 ==
  In1 : Inport
  IGBT/Diode1 : spsIGBTDiodeLib/IGBT//Diode  Ron=1e-3  Rs=1e8  Cs=inf  Measurements=off
  IGBT/Diode2 : spsIGBTDiodeLib/IGBT//Diode  Ron=1e-3  Rs=1e8  Cs=inf  Measurements=off
  NOT3 : Logic  Operator=NOT  IconShape=distinctive  AllPortsSameDT=off  OutDataTypeStr=boolean
  Series RLC Branch4 : spsSeriesRLCBranchLib/Series RLC Branch  LConnTagsString=__new0  RConnTagsString=__new0  BranchType=C  Resistance=R  Inductance=L  SetiL0=off  InitialCurrent=0  Capacitance=C  Setx0=on  InitialVoltage=Vcap0  Measurements=None
  T1 : PMIOPort  Tag=PMCPort  Side=Left
  T2 : PMIOPort  Tag=PMCPort  Port=2  Side=Left
  T3 : PMIOPort  Tag=PMCPort  Port=3  Side=Left
  wires:
  In1/1 -> IGBT/Diode1/1, NOT3/1
  NOT3/1 -> IGBT/Diode2/1
  connections:
  IGBT/Diode1/LConn1 -- Series RLC Branch4/LConn1 -- T2/RConn1
  T1/RConn1 -- IGBT/Diode1/RConn1 -- IGBT/Diode2/LConn1
  IGBT/Diode2/RConn1 -- Series RLC Branch4/RConn1 -- T3/RConn1

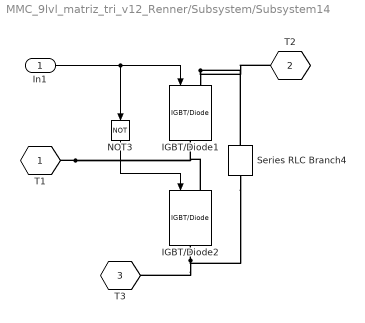
== system MMC_9lvl_matriz_tri_v12_Renner/Subsystem/Subsystem14 ==
  In1 : Inport
  IGBT/Diode1 : spsIGBTDiodeLib/IGBT//Diode  Ron=1e-3  Rs=1e8  Cs=inf  Measurements=off
  IGBT/Diode2 : spsIGBTDiodeLib/IGBT//Diode  Ron=1e-3  Rs=1e8  Cs=inf  Measurements=off
  NOT3 : Logic  Operator=NOT  IconShape=distinctive  AllPortsSameDT=off  OutDataTypeStr=boolean
  Series RLC Branch4 : spsSeriesRLCBranchLib/Series RLC Branch  LConnTagsString=__new0  RConnTagsString=__new0  BranchType=C  Resistance=R  Inductance=L  SetiL0=off  InitialCurrent=0  Capacitance=C  Setx0=on  InitialVoltage=Vcap0  Measurements=None
  T1 : PMIOPort  Tag=PMCPort  Side=Left
  T2 : PMIOPort  Tag=PMCPort  Port=2  Side=Left
  T3 : PMIOPort  Tag=PMCPort  Port=3  Side=Left
  wires:
  In1/1 -> IGBT/Diode1/1, NOT3/1
  NOT3/1 -> IGBT/Diode2/1
  connections:
  IGBT/Diode1/LConn1 -- Series RLC Branch4/LConn1 -- T2/RConn1
  T1/RConn1 -- IGBT/Diode1/RConn1 -- IGBT/Diode2/LConn1
  IGBT/Diode2/RConn1 -- Series RLC Branch4/RConn1 -- T3/RConn1

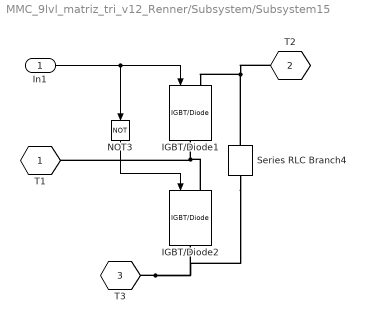
== system MMC_9lvl_matriz_tri_v12_Renner/Subsystem/Subsystem15 ==
  In1 : Inport
  IGBT/Diode1 : spsIGBTDiodeLib/IGBT//Diode  Ron=1e-3  Rs=1e8  Cs=inf  Measurements=off
  IGBT/Diode2 : spsIGBTDiodeLib/IGBT//Diode  Ron=1e-3  Rs=1e8  Cs=inf  Measurements=off
  NOT3 : Logic  Operator=NOT  IconShape=distinctive  AllPortsSameDT=off  OutDataTypeStr=boolean
  Series RLC Branch4 : spsSeriesRLCBranchLib/Series RLC Branch  LConnTagsString=__new0  RConnTagsString=__new0  BranchType=C  Resistance=R  Inductance=L  SetiL0=off  InitialCurrent=0  Capacitance=C  Setx0=on  InitialVoltage=Vcap0  Measurements=None
  T1 : PMIOPort  Tag=PMCPort  Side=Left
  T2 : PMIOPort  Tag=PMCPort  Port=2  Side=Left
  T3 : PMIOPort  Tag=PMCPort  Port=3  Side=Left
  wires:
  NOT3/1 -> IGBT/Diode2/1
  In1/1 -> NOT3/1, IGBT/Diode1/1
  connections:
  T3/RConn1 -- Series RLC Branch4/RConn1 -- IGBT/Diode2/RConn1
  IGBT/Diode2/LConn1 -- IGBT/Diode1/RConn1 -- T1/RConn1
  T2/RConn1 -- Series RLC Branch4/LConn1 -- IGBT/Diode1/LConn1

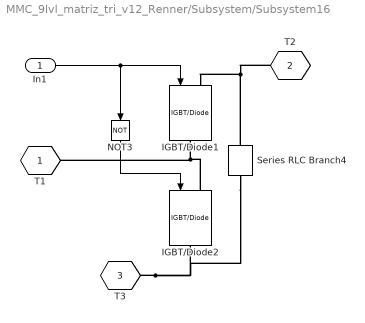
== system MMC_9lvl_matriz_tri_v12_Renner/Subsystem/Subsystem16 ==
  In1 : Inport
  IGBT/Diode1 : spsIGBTDiodeLib/IGBT//Diode  Ron=1e-3  Rs=1e8  Cs=inf  Measurements=off
  IGBT/Diode2 : spsIGBTDiodeLib/IGBT//Diode  Ron=1e-3  Rs=1e8  Cs=inf  Measurements=off
  NOT3 : Logic  Operator=NOT  IconShape=distinctive  AllPortsSameDT=off  OutDataTypeStr=boolean
  Series RLC Branch4 : spsSeriesRLCBranchLib/Series RLC Branch  LConnTagsString=__new0  RConnTagsString=__new0  BranchType=C  Resistance=R  Inductance=L  SetiL0=off  InitialCurrent=0  Capacitance=C  Setx0=on  InitialVoltage=Vcap0  Measurements=None
  T1 : PMIOPort  Tag=PMCPort  Side=Left
  T2 : PMIOPort  Tag=PMCPort  Port=2  Side=Left
  T3 : PMIOPort  Tag=PMCPort  Port=3  Side=Left
  wires:
  NOT3/1 -> IGBT/Diode2/1
  In1/1 -> NOT3/1, IGBT/Diode1/1
  connections:
  T3/RConn1 -- Series RLC Branch4/RConn1 -- IGBT/Diode2/RConn1
  IGBT/Diode2/LConn1 -- IGBT/Diode1/RConn1 -- T1/RConn1
  T2/RConn1 -- IGBT/Diode1/LConn1 -- Series RLC Branch4/LConn1

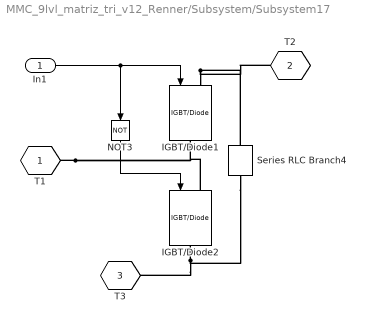
== system MMC_9lvl_matriz_tri_v12_Renner/Subsystem/Subsystem17 ==
  In1 : Inport
  IGBT/Diode1 : spsIGBTDiodeLib/IGBT//Diode  Ron=1e-3  Rs=1e8  Cs=inf  Measurements=off
  IGBT/Diode2 : spsIGBTDiodeLib/IGBT//Diode  Ron=1e-3  Rs=1e8  Cs=inf  Measurements=off
  NOT3 : Logic  Operator=NOT  IconShape=distinctive  AllPortsSameDT=off  OutDataTypeStr=boolean
  Series RLC Branch4 : spsSeriesRLCBranchLib/Series RLC Branch  LConnTagsString=__new0  RConnTagsString=__new0  BranchType=C  Resistance=R  Inductance=L  SetiL0=off  InitialCurrent=0  Capacitance=C  Setx0=on  InitialVoltage=Vcap0  Measurements=None
  T1 : PMIOPort  Tag=PMCPort  Side=Left
  T2 : PMIOPort  Tag=PMCPort  Port=2  Side=Left
  T3 : PMIOPort  Tag=PMCPort  Port=3  Side=Left
  wires:
  In1/1 -> IGBT/Diode1/1, NOT3/1
  NOT3/1 -> IGBT/Diode2/1
  connections:
  IGBT/Diode1/LConn1 -- Series RLC Branch4/LConn1 -- T2/RConn1
  T1/RConn1 -- IGBT/Diode1/RConn1 -- IGBT/Diode2/LConn1
  IGBT/Diode2/RConn1 -- Series RLC Branch4/RConn1 -- T3/RConn1

== system MMC_9lvl_matriz_tri_v12_Renner/Subsystem/Subsystem18 ==
  In1 : Inport
  IGBT/Diode1 : spsIGBTDiodeLib/IGBT//Diode  Ron=1e-3  Rs=1e8  Cs=inf  Measurements=off
  IGBT/Diode2 : spsIGBTDiodeLib/IGBT//Diode  Ron=1e-3  Rs=1e8  Cs=inf  Measurements=off
  NOT3 : Logic  Operator=NOT  IconShape=distinctive  AllPortsSameDT=off  OutDataTypeStr=boolean
  Series RLC Branch4 : spsSeriesRLCBranchLib/Series RLC Branch  LConnTagsString=__new0  RConnTagsString=__new0  BranchType=C  Resistance=R  Inductance=L  SetiL0=off  InitialCurrent=0  Capacitance=C  Setx0=on  InitialVoltage=Vcap0  Measurements=None
  T1 : PMIOPort  Tag=PMCPort  Side=Left
  T2 : PMIOPort  Tag=PMCPort  Port=2  Side=Left
  T3 : PMIOPort  Tag=PMCPort  Port=3  Side=Left
  wires:
  NOT3/1 -> IGBT/Diode2/1
  In1/1 -> NOT3/1, IGBT/Diode1/1
  connections:
  T3/RConn1 -- Series RLC Branch4/RConn1 -- IGBT/Diode2/RConn1
  IGBT/Diode2/LConn1 -- IGBT/Diode1/RConn1 -- T1/RConn1
  T2/RConn1 -- Series RLC Branch4/LConn1 -- IGBT/Diode1/LConn1

== system MMC_9lvl_matriz_tri_v12_Renner/Subsystem/Subsystem19 ==
  In1 : Inport
  IGBT/Diode1 : spsIGBTDiodeLib/IGBT//Diode  Ron=1e-3  Rs=1e8  Cs=inf  Measurements=off
  IGBT/Diode2 : spsIGBTDiodeLib/IGBT//Diode  Ron=1e-3  Rs=1e8  Cs=inf  Measurements=off
  NOT3 : Logic  Operator=NOT  IconShape=distinctive  AllPortsSameDT=off  OutDataTypeStr=boolean
  Series RLC Branch4 : spsSeriesRLCBranchLib/Series RLC Branch  LConnTagsString=__new0  RConnTagsString=__new0  BranchType=C  Resistance=R  Inductance=L  SetiL0=off  InitialCurrent=0  Capacitance=C  Setx0=on  InitialVoltage=Vcap0  Measurements=None
  T1 : PMIOPort  Tag=PMCPort  Side=Left
  T2 : PMIOPort  Tag=PMCPort  Port=2  Side=Left
  T3 : PMIOPort  Tag=PMCPort  Port=3  Side=Left
  wires:
  In1/1 -> IGBT/Diode1/1, NOT3/1
  NOT3/1 -> IGBT/Diode2/1
  connections:
  IGBT/Diode1/LConn1 -- Series RLC Branch4/LConn1 -- T2/RConn1
  T1/RConn1 -- IGBT/Diode1/RConn1 -- IGBT/Diode2/LConn1
  IGBT/Diode2/RConn1 -- Series RLC Branch4/RConn1 -- T3/RConn1

== system MMC_9lvl_matriz_tri_v12_Renner/Subsystem/Subsystem2 ==
  In1 : Inport
  IGBT/Diode1 : spsIGBTDiodeLib/IGBT//Diode  Ron=1e-3  Rs=1e8  Cs=inf  Measurements=off
  IGBT/Diode2 : spsIGBTDiodeLib/IGBT//Diode  Ron=1e-3  Rs=1e8  Cs=inf  Measurements=off
  NOT3 : Logic  Operator=NOT  IconShape=distinctive  AllPortsSameDT=off  OutDataTypeStr=boolean
  Series RLC Branch4 : spsSeriesRLCBranchLib/Series RLC Branch  LConnTagsString=__new0  RConnTagsString=__new0  BranchType=C  Resistance=R  Inductance=L  SetiL0=off  InitialCurrent=0  Capacitance=C  Setx0=on  InitialVoltage=Vcap0  Measurements=None
  T1 : PMIOPort  Tag=PMCPort  Side=Left
  T2 : PMIOPort  Tag=PMCPort  Port=2  Side=Left
  T3 : PMIOPort  Tag=PMCPort  Port=3  Side=Left
  wires:
  NOT3/1 -> IGBT/Diode2/1
  In1/1 -> NOT3/1, IGBT/Diode1/1
  connections:
  T3/RConn1 -- Series RLC Branch4/RConn1 -- IGBT/Diode2/RConn1
  IGBT/Diode2/LConn1 -- IGBT/Diode1/RConn1 -- T1/RConn1
  T2/RConn1 -- Series RLC Branch4/LConn1 -- IGBT/Diode1/LConn1

== system MMC_9lvl_matriz_tri_v12_Renner/Subsystem/Subsystem20 ==
  In1 : Inport
  IGBT/Diode1 : spsIGBTDiodeLib/IGBT//Diode  Ron=1e-3  Rs=1e8  Cs=inf  Measurements=off
  IGBT/Diode2 : spsIGBTDiodeLib/IGBT//Diode  Ron=1e-3  Rs=1e8  Cs=inf  Measurements=off
  NOT3 : Logic  Operator=NOT  IconShape=distinctive  AllPortsSameDT=off  OutDataTypeStr=boolean
  Series RLC Branch4 : spsSeriesRLCBranchLib/Series RLC Branch  LConnTagsString=__new0  RConnTagsString=__new0  BranchType=C  Resistance=R  Inductance=L  SetiL0=off  InitialCurrent=0  Capacitance=C  Setx0=on  InitialVoltage=Vcap0  Measurements=None
  T1 : PMIOPort  Tag=PMCPort  Side=Left
  T2 : PMIOPort  Tag=PMCPort  Port=2  Side=Left
  T3 : PMIOPort  Tag=PMCPort  Port=3  Side=Left
  wires:
  In1/1 -> IGBT/Diode1/1, NOT3/1
  NOT3/1 -> IGBT/Diode2/1
  connections:
  T2/RConn1 -- IGBT/Diode1/LConn1 -- Series RLC Branch4/LConn1
  T1/RConn1 -- IGBT/Diode1/RConn1 -- IGBT/Diode2/LConn1
  IGBT/Diode2/RConn1 -- Series RLC Branch4/RConn1 -- T3/RConn1

== system MMC_9lvl_matriz_tri_v12_Renner/Subsystem/Subsystem21 ==
  In1 : Inport
  IGBT/Diode1 : spsIGBTDiodeLib/IGBT//Diode  Ron=1e-3  Rs=1e8  Cs=inf  Measurements=off
  IGBT/Diode2 : spsIGBTDiodeLib/IGBT//Diode  Ron=1e-3  Rs=1e8  Cs=inf  Measurements=off
  NOT3 : Logic  Operator=NOT  IconShape=distinctive  AllPortsSameDT=off  OutDataTypeStr=boolean
  Series RLC Branch4 : spsSeriesRLCBranchLib/Series RLC Branch  LConnTagsString=__new0  RConnTagsString=__new0  BranchType=C  Resistance=R  Inductance=L  SetiL0=off  InitialCurrent=0  Capacitance=C  Setx0=on  InitialVoltage=Vcap0  Measurements=None
  T1 : PMIOPort  Tag=PMCPort  Side=Left
  T2 : PMIOPort  Tag=PMCPort  Port=2  Side=Left
  T3 : PMIOPort  Tag=PMCPort  Port=3  Side=Left
  wires:
  NOT3/1 -> IGBT/Diode2/1
  In1/1 -> NOT3/1, IGBT/Diode1/1
  connections:
  T3/RConn1 -- Series RLC Branch4/RConn1 -- IGBT/Diode2/RConn1
  IGBT/Diode2/LConn1 -- IGBT/Diode1/RConn1 -- T1/RConn1
  T2/RConn1 -- Series RLC Branch4/LConn1 -- IGBT/Diode1/LConn1

== system MMC_9lvl_matriz_tri_v12_Renner/Subsystem/Subsystem22 ==
  In1 : Inport
  IGBT/Diode1 : spsIGBTDiodeLib/IGBT//Diode  Ron=1e-3  Rs=1e8  Cs=inf  Measurements=off
  IGBT/Diode2 : spsIGBTDiodeLib/IGBT//Diode  Ron=1e-3  Rs=1e8  Cs=inf  Measurements=off
  NOT3 : Logic  Operator=NOT  IconShape=distinctive  AllPortsSameDT=off  OutDataTypeStr=boolean
  Series RLC Branch4 : spsSeriesRLCBranchLib/Series RLC Branch  LConnTagsString=__new0  RConnTagsString=__new0  BranchType=C  Resistance=R  Inductance=L  SetiL0=off  InitialCurrent=0  Capacitance=C  Setx0=on  InitialVoltage=Vcap0  Measurements=None
  T1 : PMIOPort  Tag=PMCPort  Side=Left
  T2 : PMIOPort  Tag=PMCPort  Port=2  Side=Left
  T3 : PMIOPort  Tag=PMCPort  Port=3  Side=Left
  wires:
  NOT3/1 -> IGBT/Diode2/1
  In1/1 -> NOT3/1, IGBT/Diode1/1
  connections:
  IGBT/Diode2/RConn1 -- Series RLC Branch4/RConn1 -- T3/RConn1
  IGBT/Diode2/LConn1 -- IGBT/Diode1/RConn1 -- T1/RConn1
  T2/RConn1 -- Series RLC Branch4/LConn1 -- IGBT/Diode1/LConn1

== system MMC_9lvl_matriz_tri_v12_Renner/Subsystem/Subsystem23 ==
  In1 : Inport
  IGBT/Diode1 : spsIGBTDiodeLib/IGBT//Diode  Ron=1e-3  Rs=1e8  Cs=inf  Measurements=off
  IGBT/Diode2 : spsIGBTDiodeLib/IGBT//Diode  Ron=1e-3  Rs=1e8  Cs=inf  Measurements=off
  NOT3 : Logic  Operator=NOT  IconShape=distinctive  AllPortsSameDT=off  OutDataTypeStr=boolean
  Series RLC Branch4 : spsSeriesRLCBranchLib/Series RLC Branch  LConnTagsString=__new0  RConnTagsString=__new0  BranchType=C  Resistance=R  Inductance=L  SetiL0=off  InitialCurrent=0  Capacitance=C  Setx0=on  InitialVoltage=Vcap0  Measurements=None
  T1 : PMIOPort  Tag=PMCPort  Side=Left
  T2 : PMIOPort  Tag=PMCPort  Port=2  Side=Left
  T3 : PMIOPort  Tag=PMCPort  Port=3  Side=Left
  wires:
  NOT3/1 -> IGBT/Diode2/1
  In1/1 -> NOT3/1, IGBT/Diode1/1
  connections:
  T3/RConn1 -- Series RLC Branch4/RConn1 -- IGBT/Diode2/RConn1
  IGBT/Diode2/LConn1 -- IGBT/Diode1/RConn1 -- T1/RConn1
  T2/RConn1 -- Series RLC Branch4/LConn1 -- IGBT/Diode1/LConn1

== system MMC_9lvl_matriz_tri_v12_Renner/Subsystem/Subsystem3 ==
  In1 : Inport
  IGBT/Diode1 : spsIGBTDiodeLib/IGBT//Diode  Ron=1e-3  Rs=1e8  Cs=inf  Measurements=off
  IGBT/Diode2 : spsIGBTDiodeLib/IGBT//Diode  Ron=1e-3  Rs=1e8  Cs=inf  Measurements=off
  NOT3 : Logic  Operator=NOT  IconShape=distinctive  AllPortsSameDT=off  OutDataTypeStr=boolean
  Series RLC Branch1 : spsSeriesRLCBranchLib/Series RLC Branch  LConnTagsString=__new0  RConnTagsString=__new0  BranchType=C  Resistance=R  Inductance=L  SetiL0=off  InitialCurrent=0  Capacitance=C  Setx0=on  InitialVoltage=Vcap0  Measurements=None
  T1 : PMIOPort  Tag=PMCPort  Side=Left
  T2 : PMIOPort  Tag=PMCPort  Port=2  Side=Left
  T3 : PMIOPort  Tag=PMCPort  Port=3  Side=Left
  wires:
  In1/1 -> IGBT/Diode1/1, NOT3/1
  NOT3/1 -> IGBT/Diode2/1
  connections:
  IGBT/Diode1/LConn1 -- Series RLC Branch1/LConn1 -- T2/RConn1
  T1/RConn1 -- IGBT/Diode1/RConn1 -- IGBT/Diode2/LConn1
  IGBT/Diode2/RConn1 -- Series RLC Branch1/RConn1 -- T3/RConn1

== system MMC_9lvl_matriz_tri_v12_Renner/Subsystem/Subsystem4 ==
  In1 : Inport
  IGBT/Diode1 : spsIGBTDiodeLib/IGBT//Diode  Ron=1e-3  Rs=1e8  Cs=inf  Measurements=off
  IGBT/Diode2 : spsIGBTDiodeLib/IGBT//Diode  Ron=1e-3  Rs=1e8  Cs=inf  Measurements=off
  NOT3 : Logic  Operator=NOT  IconShape=distinctive  AllPortsSameDT=off  OutDataTypeStr=boolean
  Series RLC Branch4 : spsSeriesRLCBranchLib/Series RLC Branch  LConnTagsString=__new0  RConnTagsString=__new0  BranchType=C  Resistance=R  Inductance=L  SetiL0=off  InitialCurrent=0  Capacitance=C  Setx0=on  InitialVoltage=Vcap0  Measurements=None
  T1 : PMIOPort  Tag=PMCPort  Side=Left
  T2 : PMIOPort  Tag=PMCPort  Port=2  Side=Left
  T3 : PMIOPort  Tag=PMCPort  Port=3  Side=Left
  wires:
  NOT3/1 -> IGBT/Diode2/1
  In1/1 -> NOT3/1, IGBT/Diode1/1
  connections:
  T3/RConn1 -- Series RLC Branch4/RConn1 -- IGBT/Diode2/RConn1
  IGBT/Diode2/LConn1 -- IGBT/Diode1/RConn1 -- T1/RConn1
  T2/RConn1 -- Series RLC Branch4/LConn1 -- IGBT/Diode1/LConn1

== system MMC_9lvl_matriz_tri_v12_Renner/Subsystem/Subsystem5 ==
  In1 : Inport
  IGBT/Diode1 : spsIGBTDiodeLib/IGBT//Diode  Ron=1e-3  Rs=1e8  Cs=inf  Measurements=off
  IGBT/Diode2 : spsIGBTDiodeLib/IGBT//Diode  Ron=1e-3  Rs=1e8  Cs=inf  Measurements=off
  NOT3 : Logic  Operator=NOT  IconShape=distinctive  AllPortsSameDT=off  OutDataTypeStr=boolean
  Series RLC Branch4 : spsSeriesRLCBranchLib/Series RLC Branch  LConnTagsString=__new0  RConnTagsString=__new0  BranchType=C  Resistance=R  Inductance=L  SetiL0=off  InitialCurrent=0  Capacitance=C  Setx0=on  InitialVoltage=Vcap0  Measurements=None
  T1 : PMIOPort  Tag=PMCPort  Side=Left
  T2 : PMIOPort  Tag=PMCPort  Port=2  Side=Left
  T3 : PMIOPort  Tag=PMCPort  Port=3  Side=Left
  wires:
  In1/1 -> IGBT/Diode1/1, NOT3/1
  NOT3/1 -> IGBT/Diode2/1
  connections:
  IGBT/Diode1/LConn1 -- Series RLC Branch4/LConn1 -- T2/RConn1
  T1/RConn1 -- IGBT/Diode1/RConn1 -- IGBT/Diode2/LConn1
  IGBT/Diode2/RConn1 -- Series RLC Branch4/RConn1 -- T3/RConn1

== system MMC_9lvl_matriz_tri_v12_Renner/Subsystem/Subsystem6 ==
  In1 : Inport
  IGBT/Diode1 : spsIGBTDiodeLib/IGBT//Diode  Ron=1e-3  Rs=1e8  Cs=inf  Measurements=off
  IGBT/Diode2 : spsIGBTDiodeLib/IGBT//Diode  Ron=1e-3  Rs=1e8  Cs=inf  Measurements=off
  NOT3 : Logic  Operator=NOT  IconShape=distinctive  AllPortsSameDT=off  OutDataTypeStr=boolean
  Series RLC Branch1 : spsSeriesRLCBranchLib/Series RLC Branch  LConnTagsString=__new0  RConnTagsString=__new0  BranchType=C  Resistance=R  Inductance=L  SetiL0=off  InitialCurrent=0  Capacitance=C  Setx0=on  InitialVoltage=Vcap0  Measurements=None
  T1 : PMIOPort  Tag=PMCPort  Side=Left
  T2 : PMIOPort  Tag=PMCPort  Port=2  Side=Left
  T3 : PMIOPort  Tag=PMCPort  Port=3  Side=Left
  wires:
  In1/1 -> IGBT/Diode1/1, NOT3/1
  NOT3/1 -> IGBT/Diode2/1
  connections:
  IGBT/Diode1/LConn1 -- Series RLC Branch1/LConn1 -- T2/RConn1
  T1/RConn1 -- IGBT/Diode1/RConn1 -- IGBT/Diode2/LConn1
  IGBT/Diode2/RConn1 -- Series RLC Branch1/RConn1 -- T3/RConn1

== system MMC_9lvl_matriz_tri_v12_Renner/Subsystem/Subsystem7 ==
  In1 : Inport
  IGBT/Diode1 : spsIGBTDiodeLib/IGBT//Diode  Ron=1e-3  Rs=1e8  Cs=inf  Measurements=off
  IGBT/Diode2 : spsIGBTDiodeLib/IGBT//Diode  Ron=1e-3  Rs=1e8  Cs=inf  Measurements=off
  NOT3 : Logic  Operator=NOT  IconShape=distinctive  AllPortsSameDT=off  OutDataTypeStr=boolean
  Series RLC Branch4 : spsSeriesRLCBranchLib/Series RLC Branch  LConnTagsString=__new0  RConnTagsString=__new0  BranchType=C  Resistance=R  Inductance=L  SetiL0=off  InitialCurrent=0  Capacitance=C  Setx0=on  InitialVoltage=Vcap0  Measurements=None
  T1 : PMIOPort  Tag=PMCPort  Side=Left
  T2 : PMIOPort  Tag=PMCPort  Port=2  Side=Left
  T3 : PMIOPort  Tag=PMCPort  Port=3  Side=Left
  wires:
  NOT3/1 -> IGBT/Diode2/1
  In1/1 -> NOT3/1, IGBT/Diode1/1
  connections:
  T3/RConn1 -- Series RLC Branch4/RConn1 -- IGBT/Diode2/RConn1
  IGBT/Diode2/LConn1 -- IGBT/Diode1/RConn1 -- T1/RConn1
  T2/RConn1 -- Series RLC Branch4/LConn1 -- IGBT/Diode1/LConn1

== system MMC_9lvl_matriz_tri_v12_Renner/Subsystem/Subsystem8 ==
  In1 : Inport
  IGBT/Diode1 : spsIGBTDiodeLib/IGBT//Diode  Ron=1e-3  Rs=1e8  Cs=inf  Measurements=off
  IGBT/Diode2 : spsIGBTDiodeLib/IGBT//Diode  Ron=1e-3  Rs=1e8  Cs=inf  Measurements=off
  NOT3 : Logic  Operator=NOT  IconShape=distinctive  AllPortsSameDT=off  OutDataTypeStr=boolean
  Series RLC Branch4 : spsSeriesRLCBranchLib/Series RLC Branch  LConnTagsString=__new0  RConnTagsString=__new0  BranchType=C  Resistance=R  Inductance=L  SetiL0=off  InitialCurrent=0  Capacitance=C  Setx0=on  InitialVoltage=Vcap0  Measurements=None
  T1 : PMIOPort  Tag=PMCPort  Side=Left
  T2 : PMIOPort  Tag=PMCPort  Port=2  Side=Left
  T3 : PMIOPort  Tag=PMCPort  Port=3  Side=Left
  wires:
  NOT3/1 -> IGBT/Diode2/1
  In1/1 -> NOT3/1, IGBT/Diode1/1
  connections:
  IGBT/Diode2/RConn1 -- Series RLC Branch4/RConn1 -- T3/RConn1
  IGBT/Diode2/LConn1 -- IGBT/Diode1/RConn1 -- T1/RConn1
  T2/RConn1 -- Series RLC Branch4/LConn1 -- IGBT/Diode1/LConn1

== system MMC_9lvl_matriz_tri_v12_Renner/Subsystem/Subsystem9 ==
  In1 : Inport
  IGBT/Diode1 : spsIGBTDiodeLib/IGBT//Diode  Ron=1e-3  Rs=1e8  Cs=inf  Measurements=off
  IGBT/Diode2 : spsIGBTDiodeLib/IGBT//Diode  Ron=1e-3  Rs=1e8  Cs=inf  Measurements=off
  NOT3 : Logic  Operator=NOT  IconShape=distinctive  AllPortsSameDT=off  OutDataTypeStr=boolean
  Series RLC Branch4 : spsSeriesRLCBranchLib/Series RLC Branch  LConnTagsString=__new0  RConnTagsString=__new0  BranchType=C  Resistance=R  Inductance=L  SetiL0=off  InitialCurrent=0  Capacitance=C  Setx0=on  InitialVoltage=Vcap0  Measurements=None
  T1 : PMIOPort  Tag=PMCPort  Side=Left
  T2 : PMIOPort  Tag=PMCPort  Port=2  Side=Left
  T3 : PMIOPort  Tag=PMCPort  Port=3  Side=Left
  wires:
  NOT3/1 -> IGBT/Diode2/1
  In1/1 -> NOT3/1, IGBT/Diode1/1
  connections:
  T3/RConn1 -- Series RLC Branch4/RConn1 -- IGBT/Diode2/RConn1
  IGBT/Diode2/LConn1 -- IGBT/Diode1/RConn1 -- T1/RConn1
  T2/RConn1 -- Series RLC Branch4/LConn1 -- IGBT/Diode1/LConn1
